simulink library "BalanceBtc"  (R2022b)
settings: Solver=VariableStepAuto  StartTime=0.0  StopTime=10.0  RelTol=1e-3
undefined symbols (not defined in the file or in its folder): Row
libraries: TuneVar x10, TOP x3, HandyTextFile x2, SetDsm x2, AudioStats x1, FeaturePath x1, RTC x1
settings Model: Creator=st51187  LastModifiedBy=kl13806
settings SolverCC: AlgebraicLoopSolver=TrustRegion
settings DebuggingCC: UnconnectedInputMsg=warning  UnconnectedOutputMsg=warning  UnconnectedLineMsg=warning  SFMachineParentedDataDiag=warning
settings ModelReferenceCC: EnableRefExpFcnMdlSchedulingChecks=on
settings RTWCC: DLArmComputeVersion=19.05

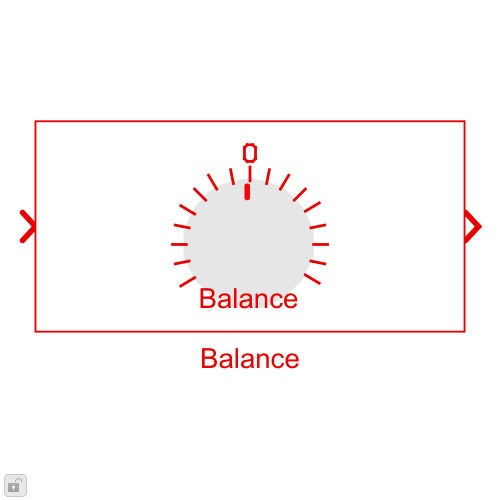
[thumbnail: Simulink's stored preview of the top-level diagram]
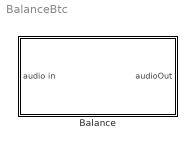
== system BalanceBtc ==
  Balance : Subsystem  mask(Blocklib Balance){FeatureName=Balance, Config=[]}
      mask prompts: FeatureName "Feature path name:"; Config "BalanceConfig"
      mask help:
      | This Balance block allows for runtime control of balancing between left and right speakers/content. Based on a gain index which comes in through a control message, channel gains for 4 different content types are computed: Left, Right, Center, and Mono.
      |
      | For the Channel to Ramper Map, enter any of the following values:
      | 1 - left channel
      | 2 - right channel
      | 3 - center channel
      | 4 - mono channel
      | -1 - unused channel (will esentially be muted)
      |
      | Enable Silent Extreme if the desired outcome when accepting an index of 0 (hard left) or 255 (hard right) should completely mute the opposing channel.
      |
      | If Silent Extreme Mutes Bass is enabled, then all mono channels will be muted, when Silent Extreme is activated.
      |
      | If this block is being used in conjunction with a stand-alone Sleeping Beauty block, disable the two Silent Extreme options.
      mask init:
      | blkh=gcbh;
      | Config=BTConfig.Assert(blkh,Config);
      | 
      | BTConfig.InitSetFeatureIfPresent(blkh,'FeatureName');
      | Config.Validate();
      | 
      | % Mask init code
      | BalanceMask.Init(blkh);
      | 
      | % Flatten config for MFBs
      | MaskNumRampers = Config.NumRampers;
      | MaskBlockH = blkh;
      | % Set boundary conditions (are these supposed to be BTC?)
      | rampRateBounds = [5,50000];
      | rampTimeBounds = [1,3000];
      mask Help:
      | The Balance block includes runtime control support for adjusting the balance dynamically.
      | - Channels may to be assigned to one of 4 possible rampers. Each channel needs to be assigned to a valid ramper (i.e. 1 - 4, or -1 for unused).
      | - The Index offset determines the index which corresponds to the balance being in the center position (typically 128).
      | - 'Enable silent extreme' mutes the speakers of the group whose gains are being 'cut' when at extreme indices.
      | - 'Disable boost' determines whether a boost is required or not. If selected, the maximum boost will be '1' on the linear scale ('0' in dB), otherwise he boost is calculated based on the curve (typically a maximum of 3 dB).
      | 
      | Control messages can be sent through the RTC block. The block is configured to accept a ramp time or rate (the rate has precedence) and an index which determines the gains for each channel group.
      | E.g., RTC_SIM_OBJ.AddREQ( 'BalanceSet', 0.1, [0001, <balance_index>, <ramp_db_per_second>, <ramp_milliseconds>, <subwoofer_index>, <surround_volume_index>]);
      | E.g., RTC_SIM_OBJ.AddREQ( 'BalanceSet', 0.1, [0001, 255, 0, 50, 128, 192]);
      mask TypeOptions FeatureName: FeaturePath/FeatureName
      mask Callback Config: BTConfig.CallbackHideIfPresent(gcbh,{'FeatureName'});
      mask Display:
      | [path,w,h] = IconBalanceMask();
      | 
      | % work in pixels since the icon does not scale
      | pos = get(gcbh,'position');
      | bw = pos(3) - pos(1);
      | bh = pos(4) - pos(2);
      | 
      | % Draw centered icon
      | xAdj = bw/2 - w/2;
      | yAdj = bh/2 - h/2;
      | for i=1:length(path)
      |     if (path(i).rgb(1) >= 0)
      |         patch(path(i).x+xAdj, path(i).y+yAdj, path(i).rgb);
      |     end
      |     if (path(i).stroke(1) >= 0)
      |         plot(path(i).x+xAdj, path(i).y+yAdj);
      |     end
      | end
      | 
      | % place feature name text
      | text(bw*0.5, 0, [FeatureName '\n\n'], 'horizontalAlignment', 'center');

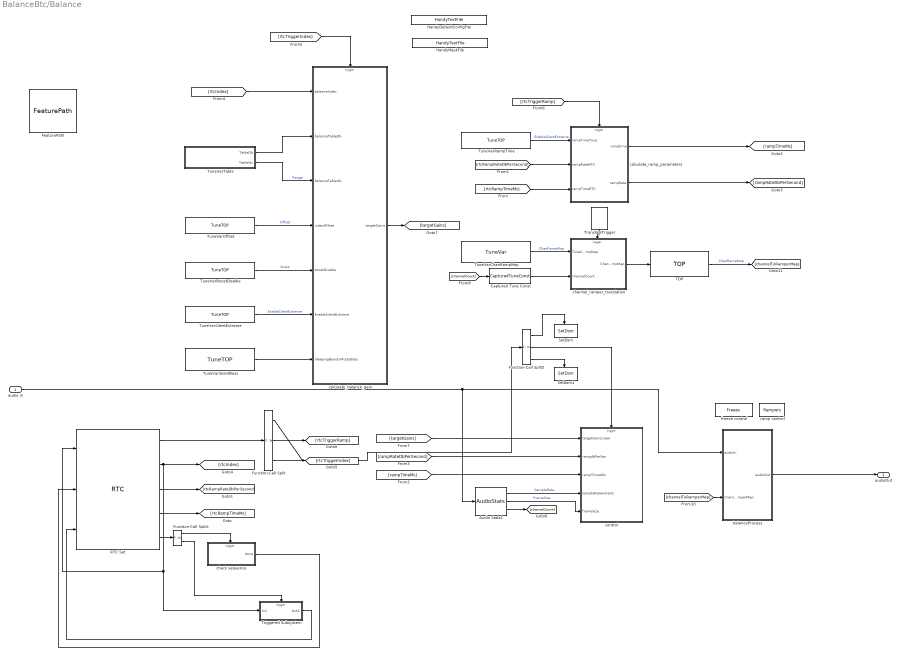
== system BalanceBtc/Balance ==
  audio in : Inport
  Audio Stats1 : AudioStats/AudioStats  DoSampleRate=on  TypeSampleRate=Inherit: auto  DoCallRate=off  TypeCallRate=Inherit: auto  DoFrameSize=on  TypeFrameSize=Inherit: auto  DoChannelCount=on  TypeChannelCount=Inherit: auto  DoTaskRateFactor=off  TypeTaskRateFactor=Inherit: auto  MacroNameRoot=AUDIO  MacroNameRootEval='AUDIO'  IsMacroNameEval=off  MacroSampleRate=off  MacroCallRate=off  MacroFrameSize=off  MacroChannelCount=off  MacroTaskRateFactor=off  MacroTaskId=off  ValidateSampleRate=off  ValueSampleRate=44100  ValidateCallRate=off  ValueCallRate=[]  ValidateFrameSize=off  ValueFrameSize=32  ValidateChannelCount=off  ValueChannelCount=[]  ValidateTaskRateFactor=off  ValueTaskRateFactor=[]
      settings: SourceProductName=Bose Talaria
  Captured Tune Const : TuneVar/CapturedTuneConst  TriggerInit=[700 257 800 293]  Role=Automatic
      settings: SourceProductName=Bose Talaria
  FeaturePath : FeaturePath/FeaturePath  FeatureName=Balance  IsGroup=off  GroupNumber=-1  IsModule=off  TriggerInit=[-435 -186 -320 -79]
      settings: SourceProductName=Bose Talaria
  Function-Call Split : FunctionCallSplit  IconShape=distinctive  NumOutputPorts=3
  Function-Call Split1 : FunctionCallSplit  IconShape=distinctive  NumOutputPorts=2  OutputPortLayout=default
  Function-Call Split2 : FunctionCallSplit  IconShape=distinctive  NumOutputPorts=3  OutputPortLayout=default
  HandyDefaultConfigFile : HandyTextFile/HandyTextFile  TemplateSource=Config  FileSuffix=Init  OpenDialogOnLoad=off  UseThisBlockName=off  AddGrandParentNamePrefix=off  TheDefaultText=|  ShowInLibBrowser=on
      | % $(FILENAME) Setup model parameters for each "Init" callback (e.g. update diagram)
      | sample_rate_in_hertz = 44100;
      | frame_size = 32;
      | sysin_channel_count = 2;
      settings: SourceProductName=Bose Talaria
  HandyMaskFile : HandyTextFile/HandyTextFile  TemplateSource=<dialog fields>  FileSuffix=Mask  OpenDialogOnLoad=off  UseThisBlockName=off  AddGrandParentNamePrefix=off  TheDefaultText=|  ShowInLibBrowser=on
      | % $(FILENAME) Setup model parameters for each "Init" callback (e.g. update diagram)
      | sample_rate_in_hertz = 44100;
      | frame_size = 32;
      | sysin_channel_count = 2;
      settings: SourceProductName=Bose Talaria
  RTC Set : RTC/RTC  REQ_Priority=RTC_Mask.NormalPriority  RequestAtInit=off  EnableRequest=on  REQElemName1=gain_index  REQElemType1=uint32  REQElemWidth1=1  REQElemInitial1=[]  REQElemName2=ramp_db_per_second  REQElemType2=uint32  REQElemWidth2=1  REQElemInitial2=[]  REQElemName3=ramp_milliseconds  REQElemType3=uint32  REQElemWidth3=1  REQElemInitial3=[]  REQElemType4=uint32  REQElemWidth4=1  REQElemInitial4=[]  REQElemType5=uint32  REQElemWidth5=1  REQElemInitial5=[]  REQElemType6=uint32  REQElemWidth6=1  REQElemInitial6=[]  REQElemType7=uint32  REQElemWidth7=1  REQElemInitial7=[]  REQElemType8=uint32  REQElemWidth8=1  REQElemInitial8=[]  REQElemType9=uint32  REQElemWidth9=1  REQElemInitial9=[]  REQElemType10=uint32  REQElemWidth10=1  REQElemInitial10=[]  EnableResponse=on  EnableRSP_StatusIn=off  RSPElemName1=gain_index  RSPElemType1=uint32  RSPElemWidth1=1  RSPElemType2=uint32  RSPElemWidth2=1  RSPElemType3=uint32  RSPElemWidth3=1  RSPElemType4=uint32  RSPElemWidth4=1  RSPElemType5=uint32  RSPElemWidth5=1  RSPElemType6=uint32  RSPElemWidth6=1  RSPElemType7=uint32  RSPElemWidth7=1  RSPElemType8=uint32  RSPElemWidth8=1  RSPElemType9=uint32  RSPElemWidth9=1  RSPElemType10=uint32  RSPElemWidth10=1  EnableNotification=on  EnableNTF_PrepTrig=off  NTFElemName1=gain_index  NTFElemType1=uint32  NTFElemWidth1=1  NTFElemType2=uint32  NTFElemWidth2=1  NTFElemType3=uint32  NTFElemWidth3=1  NTFElemType4=uint32  NTFElemWidth4=1  NTFElemType5=uint32  NTFElemWidth5=1  NTFElemType6=uint32  NTFElemWidth6=1  NTFElemType7=uint32  NTFElemWidth7=1  NTFElemType8=uint32  NTFElemWidth8=1  NTFElemType9=uint32  NTFElemWidth9=1  NTFElemType10=uint32  NTFElemWidth10=1  MaskMessageName=Set
      settings: SourceProductName=Bose Talaria
  SetDsm : SetDsm/SetDsm  DataStoreName=Freeze  Value=uint32(1)
      settings: SourceProductName=Bose Talaria
  SetDsm1 : SetDsm/SetDsm  DataStoreName=Freeze  Value=uint32(0)
      settings: SourceProductName=Bose Talaria
  TOP : TOP/TOP  TriggerInit=[1095 215 1240 275]  TopName=ChanRampMap  DataType=single  BankNumber=0  PreOverlay=false  PostOverlay=false  Role=Automatic
      settings: SourceProductName=Bose Talaria
  TranslateTrigger : TuneVar/TranslateTrigger  TriggerInit=[951 105 989 160]
      settings: SourceProductName=Bose Talaria
  Triggered Subsystem : Subsystem  TreatAsAtomicUnit=on
  TuneVarBoostDisable : TuneVar/TuneTOP  Description=Specifies the 'boost' value to be applied to the channels towards which the balance is moved. A value of '1' indicates no 'boost' (0 dB) ,whereas '0' indicates that the 'boost' must be computed from the 'cut' value (which gets computed from the Balance table). In order to preserve the overall energy, the following formula is used: Boost^2 + Cut^2 = 2.  TriggerInit=[-50 240 120 280]  TopName=BoostDisable  TuneName=BoostDisable  DataType=single  TunabilityNumber=2  MinValue=[]  MaxValue=[]  BankNumber=Config.BankNumber  PreOverlay=false  PostOverlay=false  UseSameName=on  MaskValue=Config.DefaultMaskBoostDisable
      settings: SourceProductName=Bose Talaria
  TuneVarChanRampMap : TuneVar/TuneVar  Description=|  TuneName=ChanRampMap  SpecifyMaxSize=off  VariableDim=1 (Row)  MaxSize=[1 1]  TunabilityNumber=2  MinValue=[]  MaxValue=[]  TriggerInit=[630 190 800 240]  MaskValue=Config.DefaultMaskChanRampMap
      | Specifies the ramper to which each channel is mapped. Replace the channel number with:
      | '1' - 'Right'; '2' - 'Left'; '3' - 'Center'. Currently, the 'Center' group is assigned a linear gain of 1.
      settings: SourceProductName=Bose Talaria
  TuneVarOffset : TuneVar/TuneTOP  Description=Defines the index at which the Balance is at the center i.e., neither towards the left or right sides.  TriggerInit=[-50 130 120 170]  TopName=Offset  TuneName=Offset  DataType=single  TunabilityNumber=3  MinValue=[]  MaxValue=[]  BankNumber=Config.BankNumber  PreOverlay=false  PostOverlay=false  UseSameName=on  MaskValue=Config.DefaultMaskOffset
      settings: SourceProductName=Bose Talaria
  TuneVarRampTime : TuneVar/TuneTOP  Description=Specifies the default ramp time for the rampers.  TriggerInit=[630 -80 800 -40]  TopName=RampTime  TuneName=RampTime  DataType=single  TunabilityNumber=2  MinValue=[]  MaxValue=[]  BankNumber=Config.BankNumber  PreOverlay=false  PostOverlay=false  UseSameName=on  MaskValue=30
      settings: SourceProductName=Bose Talaria
  TuneVarSilentBass : TuneVar/TuneTOP  TriggerInit=[-50 452 120 508]  TopName=SleepingBeautyMutesBass  TuneName=SleepingBeautyMutesBass  DataType=single  TunabilityNumber=1  MinValue=[]  MaxValue=[]  BankNumber=Config.BankNumber  PreOverlay=false  PostOverlay=false  UseSameName=on  MaskValue=Config.DefaultMaskSilentExtremeBass
      settings: SourceProductName=Bose Talaria
  TuneVarSilentExtreme : TuneVar/TuneTOP  Description=|  TriggerInit=[-50 350 120 390]  TopName=EnableSilentExtreme  TuneName=EnableSilentExtreme  DataType=single  TunabilityNumber=2  MinValue=[]  MaxValue=[]  BankNumber=Config.BankNumber  PreOverlay=false  PostOverlay=false  UseSameName=on  MaskValue=Config.DefaultMaskSilentExtreme
      | 0 implies no special handling
      | 1 implies special muting of the "cut" channel, in addition to the center channels) when the input control is at its extremes (lowest or highest index is provided)
      settings: SourceProductName=Bose Talaria
  TuneVarTable : Subsystem  Description=Given in dB, sets the maximum impact of balance processing among channels.
  balanceProcess : MATLAB Function  TreatAsAtomicUnit=on
  calculate_balance_gain : MATLAB Function  TreatAsAtomicUnit=on
  calculate_ramp_parameters : MATLAB Function  TreatAsAtomicUnit=on
  channel_ramper_translation : MATLAB Function  TreatAsAtomicUnit=on
  check sequence : MATLAB Function  TreatAsAtomicUnit=on
  control : MATLAB Function  TreatAsAtomicUnit=on
  freeze control : DataStoreMemory  DataStoreName=Freeze  EmbeddedSignalClassName=Bose.Signal  ShowAdditionalParam=off  OutDataTypeStr=uint32
  ramp control : DataStoreMemory  DataStoreName=Rampers  InitialValue=Config.DlgRamperInit  EmbeddedSignalClassName=Bose.Signal  ShowAdditionalParam=off  OutDataTypeStr=Bus: rgain_bus
  audioOut : Outport  VectorParamsAs1DForOutWhenUnconnected=off
  wires:
  Function-Call Split/2 -> [rtcTriggerRamp]
  Function-Call Split/1 -> [rtcTriggerIndex]
  [rtcIndex] -> calculate_balance_gain/1(balanceIndex)
  Captured Tune Const/1 -> channel_ramper_translation/2(channelCount)
  [channelCount] -> Captured Tune Const/1
  Audio Stats1/3 -> [channelCount]
  TOP/1 -> [channelToRamperMap]  "ChanRampMap"
  TuneVarChanRampMap/1 -> channel_ramper_translation/1(TuneChanRampMap)  "ChanRampMap"
  channel_ramper_translation/1(ChanRampMap) -> TOP/1
  TranslateTrigger/1 -> channel_ramper_translation/Trigger
  TuneVarTable/1(TableDb) -> calculate_balance_gain/2(balanceTableDb)
  [channelToRamperMap] -> balanceProcess/2(channelToRamperMap)
  Audio Stats1/1 -> control/4(sampleRateInHertz)  "SampleRate"
  [rampRateDbPerSecond] -> control/2(rampdbPerSec)
  [targetGains] -> control/1(targetGainLinear)
  [rampTimeMs] -> control/3(rampTimesMs)
  Function-Call Split/3 -> Function-Call Split2/1
  audio in/1 -> Audio Stats1/1, balanceProcess/1(audioIn)
  Audio Stats1/2 -> control/5(frameSize)  "FrameSize"
  balanceProcess/1(audioOut) -> audioOut/1
  calculate_balance_gain/1(targetGains) -> [targetGains]
  [rtcTriggerRamp] -> calculate_ramp_parameters/Trigger
  [rtcTriggerIndex] -> calculate_balance_gain/Trigger
  RTC Set/2 -> Triggered Subsystem/1(In1), RTC Set/1, [rtcIndex]
  calculate_ramp_parameters/2(rampRate) -> [rampRateDbPerSecond]
  calculate_ramp_parameters/1(ramptime) -> [rampTimeMs]
  [rtcRampRateDbPerSecond] -> calculate_ramp_parameters/2(rampRateRTC)
  [rtcRampTimeMs] -> calculate_ramp_parameters/3(rampTimeRTC)
  TuneVarRampTime/1 -> calculate_ramp_parameters/1(rampTimeTune)  "EnableSilentExtreme"
  RTC Set/3 -> [rtcRampRateDbPerSecond]
  RTC Set/4 -> [rtcRampTimeMs]
  RTC Set/1 -> Function-Call Split/1
  TuneVarOffset/1 -> calculate_balance_gain/4(indexOffset)  "Offset"
  TuneVarSilentExtreme/1 -> calculate_balance_gain/6(EnableSilentExtreme)  "EnableSilentExtreme"
  TuneVarTable/2(TableIdx) -> calculate_balance_gain/3(balanceTableIdx)  "Range"
  TuneVarBoostDisable/1 -> calculate_balance_gain/5(boostDisable)  "Scale"
  check sequence/1(done) -> RTC Set/2
  RTC Set/5 -> Function-Call Split1/1
  Function-Call Split1/1 -> check sequence/Trigger
  Function-Call Split1/2 -> Triggered Subsystem/Trigger
  Triggered Subsystem/1(Out1) -> RTC Set/3
  TuneVarSilentBass/1 -> calculate_balance_gain/7(SleepingBeautyMutesBass)
  Function-Call Split2/2 -> control/Trigger
  Function-Call Split2/3 -> SetDsm1/Trigger
  Function-Call Split2/1 -> SetDsm/Trigger

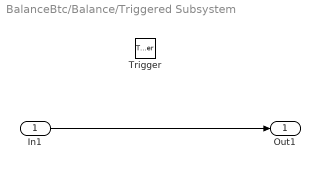
== system BalanceBtc/Balance/Triggered Subsystem ==
  In1 : Inport
  Trigger : TriggerPort  TriggerType=function-call  VariantControl=Variant
  Out1 : Outport
  wires:
  In1/1 -> Out1/1

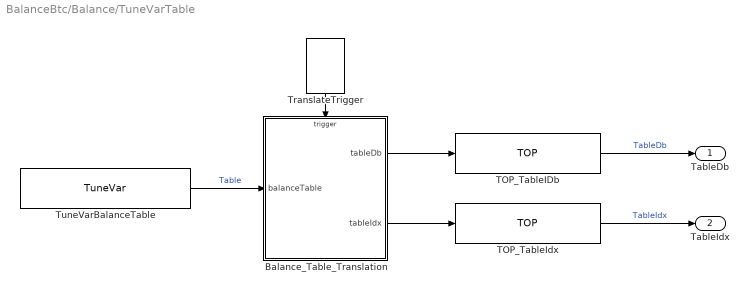
== system BalanceBtc/Balance/TuneVarTable ==
  Balance_Table_Translation : MATLAB Function  TreatAsAtomicUnit=on
  TOP_TableIDb : TOP/TOP  TriggerInit=[455 -5 600 35]  TopName=TableDb  DataType=single  BankNumber=0  PreOverlay=false  PostOverlay=false  Role=Automatic
      settings: SourceProductName=Bose Talaria
  TOP_TableIdx : TOP/TOP  TriggerInit=[455 65 600 105]  TopName=TableIdx  DataType=single  BankNumber=Config.BankNumber  PreOverlay=false  PostOverlay=false  Role=Automatic
      settings: SourceProductName=Bose Talaria
  TranslateTrigger : TuneVar/TranslateTrigger  TriggerInit=[306 -100 344 -45]
      settings: SourceProductName=Bose Talaria
  TuneVarBalanceTable : TuneVar/TuneVar  Description=Define the balance curve using a table, with the first column being the list of indices and the second column being the corresponding balance gains in dB. Gain values for indices in between the elements in the table are linearly interpolated.  TuneName=Table  SpecifyMaxSize=on  VariableDim=1 (Row)  MaxSize=[30 2]  TunabilityNumber=3  MinValue=0  MaxValue=[]  TriggerInit=[20 30 190 70]  MaskValue=[[0,10,31,52,74,95,116,128,138,159,180,202,223,244,255];[-30,-27,-14,-7,-5,-3,-1,0,-1,-3,-5,-7,-14,-27,-30]]'
      settings: SourceProductName=Bose Talaria
  TableDb : Outport  VectorParamsAs1DForOutWhenUnconnected=off
  TableIdx : Outport  Port=2  VectorParamsAs1DForOutWhenUnconnected=off
  wires:
  TOP_TableIDb/1 -> TableDb/1  "TableDb"
  Balance_Table_Translation/1(tableDb) -> TOP_TableIDb/1
  TranslateTrigger/1 -> Balance_Table_Translation/Trigger
  Balance_Table_Translation/2(tableIdx) -> TOP_TableIdx/1
  TuneVarBalanceTable/1 -> Balance_Table_Translation/1(balanceTable)  "Table"
  TOP_TableIdx/1 -> TableIdx/1  "TableIdx"

== matlab function BalanceBtc/Balance/check sequence ==
  data: done output; Rampers data_store_memory; MaskNumRampers parameter
  events: trigger input FUNCTION_CALL_EVENT
function done = GetCompletedSequence(MaskNumRampers)
% Function which checks if the notification sequence
% has completed successfully 

global Rampers;

% Assume the work is complete until proven otherwise
done = true;

for i=1:MaskNumRampers
   if (Rampers(i).targetGain ~= Rampers(i).currentGain)
       done = false; % just proved otherwise
       break;
   end
end

== matlab function BalanceBtc/Balance/control ==
  data targetGainLinear settings: description=This vector signal must provide a linear target gain for every ramper.
  data rampdbPerSec settings: description="If provided (i.e. non zero), this argument causes the \"ramp times (ms)\" input to be ignored. The block will calculate ramp times itself to ensure all gain changes happen at the db_per_sec slope provided."
  data rampTimesMs settings: description=|
      | The rampTimes_ms signal can accept one or more ramp times. If only one time is given, it is applied to all rampers. When more than one time is given, the times are delt out to the rampers in order. If not enough times are specified to cover all the rampers, the last given time is filled in to any remaining rampers.
      | NOTE: this input signal is entirely ignored if the db_per_sec input signal is non-zero. Attach the db_per_sec input to a ground block if you want to provide ramp times via this input.
  data sampleRateInHertz settings: description="This input is required for control calculations to work. The \"Audio Stats\" block is a handy tool to lift this property right off an inbound audio signal and feed it to this block automatically without using workspace parameters or other constants."
  data frameSize settings: description="This input is required for control calculations to work. The \"Audio Stats\" block is a handy tool to lift this property right off an inbound audio signal and feed it to this block automatically without using workspace parameters or other constants."
  data: targetGainLinear input size=[1 MaskNumRampers]; rampdbPerSec input; rampTimesMs input; sampleRateInHertz input; frameSize input; Rampers data_store_memory; MaskNumRampers parameter
  events: trigger input FUNCTION_CALL_EVENT
function control(...
     targetGainLinear, rampdbPerSec, rampTimesMs, sampleRateInHertz, ...
     frameSize, ... % inputs
     MaskNumRampers) % parameters
%#codegen
% CONTROL LOGIC:
% Shift of 'balance' between the 'Right' and 'Left' channel groups is
% achieved by multiplying the corresponding 'cut' or 'boost' gain. As the
% index increases from 0, the balance shifts from left to right. Channels
% corresponding to the 'center' group are not modified. 
% rampdbPerSec takes precidence:
% If dbPerSec has a non-zero value then any ramp_times_ms values are
% ignored and the dbPerSec is used to determine ramper timing.
% Inputs:
%   targetGainLinear: Indicates the gain (in linear scale) which needs to
%       be applied to the audio. Gain values can be mapped to the ramper
%       configuration.
%   rampTimeMs: Indicates the time in milliseconds in which the gain of the
%       rampers must change from their current to target values.
%   rampdbPerSecond: Indicates the rate in dB/second at which the gain of the
%       rampers must change from their current to target values. If this
%       value is non-zero, it is used to compute the ramp time and
%       'rampTimeMs' is discarded (if specified).
%   rgain_SILENT_GAIN: Parameter defined in the initFcn callback.

% Control Data:
%   Freeze(1) freezes the processing during this control operation
%   Rampers(1) is the ramper for the 'Left' group. Boost vs. cut 
%        is determined by the value of the balance index.
%   Rampers(2) is the ramper for the 'Right' group. Boost vs. cut is determined by
%        the value of the balance index.
%   Rampers(3) is the ramper for the 'Center' group. Boost vs. cut is determined by
%        the value of the balance index.
%   Rampers(4) is the ramper for the 'Mono' group (supporting "Sleeping
%       Beauty Mutes Bass"). Boost vs. cut is determined by the value of 
%       the balance index.

global Rampers;

% Step 1: FREEZE the gain ramper so that we can perform calculations based
% on the current gain value. (This step is done outside on canvas now)

% This block replaces much of rgainy, but uses its own silent gain value.
% The reason why is not documented, but it does impact all the test cases.
% Use this special value instead of RgainBusUtil.GetSilentGainLinear
rgain_SILENT_GAIN = single(10^(-126/20));

% Step 2: Nudge the gain values a bit if they are sitting at zero.
% When this control set goes live, ensure that the current gain will move.
% If current gain is zero, replace with a value very close to zero. What we
% really want is a value which is on the edge of perception - not too small
% or large. If the value is too small, we'll waste some of our ramp time
% in perceived silence. If the value is too large, the audio will lurch
% into perceptability at the start of the ramp.
% UPDATE: This will now loop over 4 rampers

currentGainLinear = zeros(1,MaskNumRampers,'single');
for i = 1:MaskNumRampers
    currentGainLinear(i) = max(Rampers(i).currentGain, rgain_SILENT_GAIN);
    targetGainLinear(i) = max(targetGainLinear(i), rgain_SILENT_GAIN);
end

% Step 3a: If a slope in dB/second is provided, ignore the ramp time
% and instead calculate a new ramp time that matches the slope.
rampMs = zeros(1,MaskNumRampers,'single');
if (rampdbPerSec)
    currentGainDb = 20*log10(currentGainLinear);
    targetGainDb = 20*log10(targetGainLinear);
    diff = abs(currentGainDb - targetGainDb);
    rampMs = diff / single(rampdbPerSec) * 1000;
else
    rampMs(:) = single(rampTimesMs);
end
    
% Step 3b: QUANTIZE the desired ramp time to our FrameSize. Also retrieve 
% the whole number of frames required to best match requested ramp time.
% Ensure that at least one frame is used. The frame size will therefore
% determine the steepest ramp (i.e. within one frame you can go anywhere).
quantumMs = 1000 * frameSize / sampleRateInHertz;
numFrames = rampMs / quantumMs;
numFrames = max (1, ceil(numFrames));
quantizedRampTimeMs = numFrames * quantumMs;

% UPDATE: Loop over 4 rampers now (L, R, C, and Mono)
for ramper=1:MaskNumRampers
    % In order to have the desired ramp time, the slope must vary dependent
    % on the gain differencebetween target and current value.
    % Ramper's coefficient is therefore calculated as follows:
    %
    %   TargetGain = CurrentGain *( RampCoef ^ (Fs*RampTime_ms/1000) )
    %
    % therefore...
    %
    %                     log(TargetGain/CurrentGain)
    %   log(RampCoef) = ------------------------------
    %                        Fs*(RampTime_ms/1000)
    %
    factor = log( targetGainLinear(ramper) / currentGainLinear(ramper) );
    RampCoef = double(exp(factor / (sampleRateInHertz * quantizedRampTimeMs(ramper) / 1000)));
    
    % Output control signals
    Rampers(ramper).frameCount  = int32(numFrames(ramper));    
    Rampers(ramper).targetGain  = targetGainLinear(ramper);
    Rampers(ramper).rampCoeff = single(RampCoef);
    Rampers(ramper).currentGain = currentGainLinear(ramper);
end
% unfreeze the gain (This step is done outside on canvas now)

== matlab function BalanceBtc/Balance/channel_ramper_translation ==
  data: ChanRampMap output; TuneChanRampMap input; channelCount input; MaskNumRampers parameter
  events: trigger input FUNCTION_CALL_EVENT
function ChanRampMap  = fcn(TuneChanRampMap, channelCount, ... % inputs
    MaskNumRampers) % parameters

% Verifies if each channel is assigned to one of the 4 possible rampers. 
% Acceptable rampers:
% 1: left
% 2: right
% 3: center
% 4: unused

argName = 'Balance';

% Ensure each channel is present in the map
inputMapWidth = numel(TuneChanRampMap.Value);
if (inputMapWidth ~= channelCount)
   error(['Error in %s : Channel-to-ramper map width [%d] does not match number of ',...
       'audio channels [%d]. Make sure all channels are assigned ',...
       'to either the left or right groups.'], argName, inputMapWidth, ...
       channelCount);
end

% Verify that the channels are assigned to valid group numbers.

if (numel(unique(TuneChanRampMap.Value)) > (MaskNumRampers + 1))
    error(['Error in [%s] : Atleast 1 channel has been assigned to the incorrect group.' ...
        'Group numbers assigned to channels in the Channel-to-ramper '...
        'map should be a number between 1 and 4, corresponding to one '...
        'of the 4 possible speaker contents .'], argName);        
end

if (sum(TuneChanRampMap.Value == 0) > 0)
   error(['Error in [%s] : Valid ramper values for the channel to '...
       'ramper map must be between 1 and 4, or "-1" to indicate an '... 
       'unused channel .'], argName);
end

ChanRampMap = int32(TuneChanRampMap.Value);

== matlab function BalanceBtc/Balance/TuneVarTable/Balance_Table_Translation ==
  data: tableDb output; tableIdx output; balanceTable input
  events: trigger input FUNCTION_CALL_EVENT
function [tableDb, tableIdx] = fcn(balanceTable)
%#codegen

% Set up the size and datatype of our TOP outputs:
maxTableSize = numel(balanceTable.Value) / 2;
idxType = 'uint8';
idxStorageType = 'uint32';
dbType = 'single';
tableIdx = zeros(1,maxTableSize,idxStorageType);
tableDb = zeros(1,maxTableSize,dbType);

% separate the pairs into their index and value components
givenPairs = balanceTable.Size(1);
indexes = balanceTable.Value(1:givenPairs,1);
values = balanceTable.Value(1:givenPairs,2);

% then sort and ignore duplicates
[cleanIdx,map] = unique(indexes);

% Validate input sizes
numPairs = numel(map);
argName='BalanceTable';

% Validate: enough data?
if (numPairs < 2)
    TranslateError('%s must have at least 2 index pairs. Encounted value with only %f pairs\n', argName, numPairs);
end

% Validate: Highest index still below 255?
if (cleanIdx(1) < 0 || cleanIdx(end) > intmax(idxType))
    TranslateError('%s out of range table index %f encountered. Index must be between 0 and %d.\n',argName,cleanIdx(end),intmax(idxType));
end

% fill in the table buffer with provided pairs
tableIdx(1:numPairs) = cleanIdx(1:numPairs);
tableDb(1:numPairs) = values(map(1:numPairs));

% fill the rest of the table buffer with the last entry
remainingPairs = numel(map)+1:maxTableSize;
tableIdx(remainingPairs) = tableIdx(numPairs);
tableDb(remainingPairs) =  tableDb(numPairs);

end

== matlab function BalanceBtc/Balance/balanceProcess ==
  data: audioIn input; audioOut output; channelToRamperMap input; Rampers data_store_memory; Freeze data_store_memory; MaskNumRampers parameter
function audioOut  = balanceProcess(audioIn, channelToRamperMap, ... % inputs
    MaskNumRampers)  % parameters

% Applies the Left and Right gains to the respective channels via multiple
%   rampers
% Inputs:
%  audioIn: Input audio
%  channelToRamperMap: Input channels mapped to their corresponding ramper.
%  MaskNumRampers: Number of rampers (set in the Mask file) = 4

% Data Store objects (registered in "Edit Data" dialog)
global Rampers;
global Freeze;

% Figure out the frame size, channel count and number of rampers
[frameSize, ~] = size(audioIn);

% set the size and datatype of the output buffer
audioOut = coder.nullcopy(audioIn);

%   Every channel needs a ramper, but every ramper does not need to be on a
%   channel necessarily.
for ramper = 1:MaskNumRampers
    % Get the gains
    gain = Rampers(ramper).currentGain;
    rampCoeffMultipliers = ones(1, frameSize, 'single');
    if (Freeze(1) == false)
        if (Rampers(ramper).frameCount == 0)
            % The ramp is finished. Stop ramping and SNAP to the target
            gain = Rampers(ramper).targetGain;
        else
            % The ramp is *NOT* frozen or done: gain is moving
            k = Rampers(ramper).rampCoeff;
            rampCoeffMultipliers = (k * rampCoeffMultipliers) .^ (1:frameSize);
            Rampers(ramper).frameCount = Rampers(ramper).frameCount - 1;
        end
    end
    
    % Apply the gains to the corresponding channels via the Mask parameter
    % and tuneTop paramter "channelToRamperMap".  
    currentChannelGroup = find(channelToRamperMap == ramper);
    for ch = 1:numel(currentChannelGroup)
        audioOut(:,currentChannelGroup(ch)) = (gain * rampCoeffMultipliers)' .* audioIn(:,currentChannelGroup(ch));
    end
    Rampers(ramper).currentGain = gain * rampCoeffMultipliers(end);
end

% If ramper value of -1 is encountered, this indicates an unused channel.
% Assign values of zero to all samples of these channels.
unusedChannelGroup = find(channelToRamperMap == -1);
for unusedCh = 1:numel(unusedChannelGroup)
    audioOut(:,unusedChannelGroup(unusedCh)) = 0;
end

== matlab function BalanceBtc/Balance/calculate_balance_gain ==
  data: balanceIndex input; balanceTableDb input; balanceTableIdx input; indexOffset input; boostDisable input; EnableSilentExtreme input; SleepingBeautyMutesBass input; targetGains output; MaskNumRampers parameter
  events: trigger input FUNCTION_CALL_EVENT
function targetGains  = Calculate_Balance_Gain(balanceIndex, ...
    balanceTableDb, balanceTableIdx, ...
    indexOffset, boostDisable, EnableSilentExtreme, SleepingBeautyMutesBass, MaskNumRampers)

% Computes the balance gains for the 'left' and 'right' channel groups. 
% Based on the position of the balance index in 'balanceTableIdx', the 
% corresponding 'cut' gain is computed from the 'balanceTableDb'. If the 
% index lies between two entries in the table, the gain is computed by 
% linear interpolation between the corresponding gain table entries. 
% The 'boost' gain is computed based from the 'cut' gain depending on the
% value of the tune variable, 'boostDisable'. If set to '1', boost is 0 dB 
% and if '0', in order to preserve energy, the boost is computed based on
% the following equation: Boost^2 + Cut^2 = 2. 
% If 'silent extreme' is enabled and the index at either extreme is
% requested, channels belonging to the group which receives a gain 'cut'
% are muted.

j = uint8(1);
cut_linear = single(0.0);

targetGains = coder.nullcopy(ones(1,MaskNumRampers,'single'));
balanceIndex = single(balanceIndex);
% random comment


% Find the left and the right gains
% Based on the balance table, the dB value of the index is calculated
while (j <= numel(balanceTableIdx))
    if (balanceIndex <= balanceTableIdx(j))
        if (j <= 1)  % first indexed value is linearly interpolated to zero
            if (balanceTableIdx(j))
                percent = balanceIndex / balanceTableIdx(j);
            else
                percent = single(1);
            end
            cut_linear = percent * 10 ^ (balanceTableDb(j) / 20);
        else         % other values are interpolated in db space
            lastIdx = single(balanceTableIdx(j-1));
            percent = (balanceIndex - lastIdx) / (balanceTableIdx(j) - lastIdx);
            cut_linear = 10 ^ (((percent * (balanceTableDb(j) - balanceTableDb(j-1))) + balanceTableDb(j-1)) / 20);
        end
        break;
    else
        j = j + 1;
    end
end

% Boost of > 0 dB is dependant on tuning. If the tune variable is SET (1),
% boost of 0 dB is applied (i.e. linear value of 1). If the tune variable
% is RESET (0), a boost of 3 dB is applied
if boostDisable == 0
    boost_linear = sqrt(2.0 - cut_linear^2);
else
    boost_linear = single(1);
end

% % if silent extreme is enabled and we're extreme, make the cut complete
% % (Sleeping Beauty)
if (EnableSilentExtreme && abs(balanceIndex - indexOffset) >= (indexOffset-1))
    cut_linear = single(0);
end

% Assign left and right Gain Values
if (balanceIndex - indexOffset) > 0 % Left speakers attenuated
    left = single(cut_linear);
    right = single(boost_linear);
else
    left = single(boost_linear);
    right = single(cut_linear);
end

% Assign remaining gain values 
center = (left + right) * 0.5;
mono = center;

% Number to Content Key
targetGains(1) = left;
targetGains(2) = right;
targetGains(3) = center;
targetGains(4) = mono;

% (Sleeping Beauty)
% if silent extreme is enabled and we're extreme, cut center freqs
if (EnableSilentExtreme && abs(balanceIndex - indexOffset) >= (indexOffset-1))
    targetGains(3) = 0;
    if (SleepingBeautyMutesBass)
        targetGains(4) = 0;
    end
end

== matlab function BalanceBtc/Balance/calculate_ramp_parameters ==
  data: rampTimeTune input; rampRateRTC input; rampTimeRTC input; ramptime output; rampRate output; rampRateBounds parameter; rampTimeBounds parameter
  events: trigger input FUNCTION_CALL_EVENT
function [ramptime, rampRate]  = calculate_ramp_parameters(...
    rampTimeTune, rampRateRTC,rampTimeRTC, ... % inputs
    rampRateBounds, rampTimeBounds) % parameters

% Ramp time and rate are provided to the block through RTC messages. However 
% in case neither of them are provided, the block will use the default ramp 
% time given in the tune variables.

    ramptime = single(rampTimeTune);
    rampRate = single(0);

    if (rampRateRTC)
        rampRate = single(rampRateRTC);
        rampRate = max(rampRateBounds(1), rampRate);
        rampRate = min(rampRateBounds(2), rampRate);
    end
    if (rampTimeRTC)
        ramptime = single(rampTimeRTC);
    end
    ramptime = max(rampTimeBounds(1), ramptime);
    ramptime = min(rampTimeBounds(2), ramptime);
end
